simulink model "Cambers"  (R2024b)
settings: Solver=VariableStepAuto  StartTime=0  StopTime=30  RelTol=1e-3
libraries: simulink x2
settings Model: Creator=owen  LastModifiedBy=owen

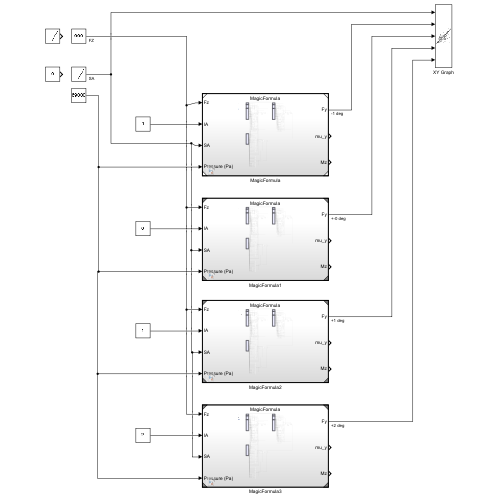
[thumbnail: Simulink's stored preview of the top-level diagram]
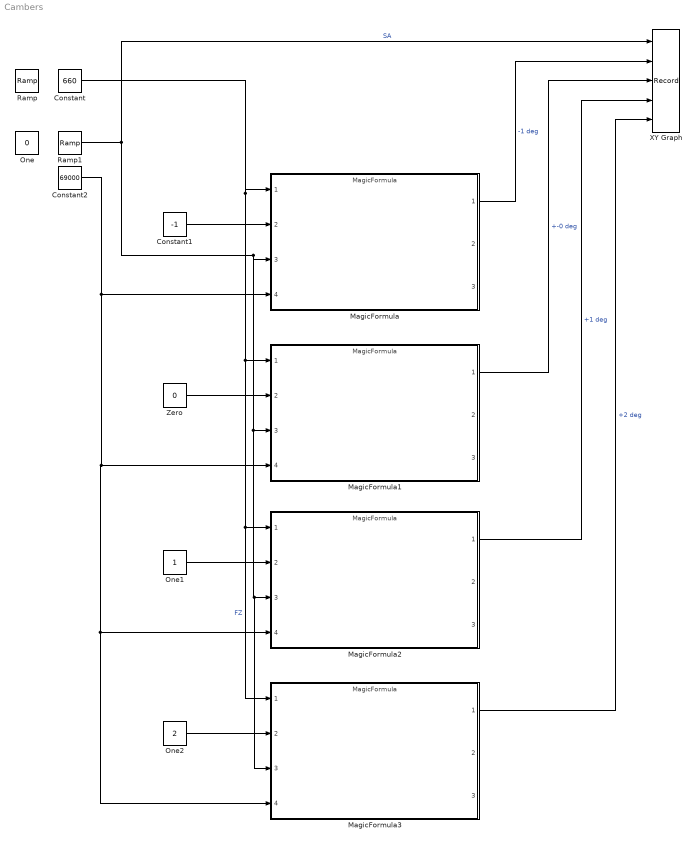
== system Cambers ==
  Constant : Constant  Value=660
  Constant1 : Constant  Value=-1
  Constant2 : Constant  Value=69000
  MagicFormula{,1..3} (4 alike) : ModelReference  ModelNameDialog=MagicFormula.slx  SimulationMode=Normal  ModelReferenceVersion=1.51
  One : Constant  Value=0  OutDataTypeStr=Inherit: Inherit via back propagation
  One1 : Constant  OutDataTypeStr=Inherit: Inherit via back propagation
  One2 : Constant  Value=2  OutDataTypeStr=Inherit: Inherit via back propagation
  Ramp : simulink/Sources/Ramp  slope=1  start=0  InitialOutput=0
  Ramp1 : simulink/Sources/Ramp  slope=1  start=0  InitialOutput=-15
  XY Graph : Record  FileSettingsInternal="{\"entries\":[{\"content\":{\"excelSettings\":{\"content\":{},\"type\":\"Streamout.ExcelSettings\"}},\"type\":\"Streamout.FileSettingStorage\",\"uuid\":\"\"}],\"packageUris\":[\"http:\\/\\/schema.mathworks.com\\/mf0\\/streamout_blocks\\/R2020a\"],\"version\":\"1.0\"}"  Layout=[1 1]  SignalsInternal="{\"entries\":[{\"content\":{\"signals\":[{\"content\":{\"blockPath\":[],\"dimensions\":[1],\"domain\":\"\",\"lineColor\":\"#a2142f\",\"plots\":[ 1 ],\"port\":1,\"sid\":[\"\"],\"signalID\":1,\"signalName\":\"SA\"},\"type\":\"RecordBlkView.Signal\",\"uuid\":\"\"},{\"content\":{\"blockPath\":[],\"dimensions\":[1],\"domain\":\"\",\"lineColor\":\"#139fff\",\"plots\":[ 1 ],\"port\":2,\"sid\":[\"\"],\"signalID\":2,\"signalName\":\"-1 deg\"},\"type\":\"RecordBlkView.Signal\",\"uuid\":\"\"},{\"content\":{\"blockPath\":[],\"dimensions\":[1],\"domain\":\"\",\"lineColor\":\"#ff6929\",\"lineWidth\":2,\"plots\":[ 1 ],\"port\":3,\"sid\":[\"\"],\"signalID\":3,\"signalName\":\"+-0 deg\"},\"type\":\"RecordBlkView.Signal\",\"uuid\":\"\"},{\"content\":{\"blockPath\":[],\"dimensions\":[1],\"domain\":\"\",\"lineColor\":\"#b746ff\",\"lineWidth\":2,\"plots\":[ 1 ],\"port\":4,\"sid\":[\"\"],\"signalID\":4,\"signalName\":\"+1 deg\"},\"type\":\"RecordBlkView.Signal\",\"uuid\":\"\"},{\"content\":{\"blockPath\":[],\"dimensions\":[1],\"domain\":\"\",\"lineColor\":\"#64d413\",\"lineWidth\":2,\"plots\":[ 1 ],\"port\":5,\"sid\":[\"\"],\"signalID\":5,\"signalName\":\"+2 deg\"},\"type\":\"RecordBlkView.Signal\",\"uuid\":\"\"}]},\"type\":\"RecordBlkView.InputSignals\",\"uuid\":\"\"}],\"packageUris\":[\"http:\\/\\/schema.mathworks.com\\/mf0\\/streamout_blocks\\/R2020a\"],\"version\":\"1.0\"}"  VisualizationBindings="{\"xyplotplugin\":{\"info\":[{\"series\":[{\"bindingParametersList\":[{\"parameter\":\"X-Axis\",\"signalID\":1,\"signalName\":\"SA\"},{\"parameter\":\"Y-Axis\",\"signalID\":2,\"signalName\":\"-1 deg\"}],\"seriesID\":0},{\"bindingParametersList\":[{\"parameter\":\"X-Axis\",\"signalID\":1,\"signalName\":\"SA\"},{\"parameter\":\"Y-Axis\",\"signalID\":3,\"signalName\":\"+-0 deg\"}],\"seriesID\":1},{\"bindingParametersList\":[{\"parameter\":\"X-Axis\",\"signalID\":1,\"signalName\":\"SA\"},{\"parameter\":\"Y-Axis\",\"signalID\":4,\"signalName\":\"+1 deg\"}],\"seriesID\":2},{\"bindingParametersList\":[{\"parameter\":\"X-Axis\",\"signalID\":1,\"signalName\":\"SA\"},{\"parameter\":\"Y-Axis\",\"signalID\":5,\"signalName\":\"+2 deg\"}],\"seriesID\":3}],\"subplotID\":1}]}}"  CompatibilityTag=XY
  Zero : Constant  Value=0  OutDataTypeStr=Inherit: Inherit via back propagation
  wires:
  Constant/1 -> MagicFormula3/1, MagicFormula2/1, MagicFormula1/1, MagicFormula/1  "FZ"
  Ramp1/1 -> XY Graph/1, MagicFormula3/3, MagicFormula2/3, MagicFormula1/3, MagicFormula/3  "SA"
  MagicFormula/1 -> XY Graph/2  "-1 deg"
  MagicFormula3/1 -> XY Graph/5  "+2 deg"
  MagicFormula2/1 -> XY Graph/4  "+1 deg"
  MagicFormula1/1 -> XY Graph/3  "+-0 deg"
  Constant1/1 -> MagicFormula/2
  Zero/1 -> MagicFormula1/2
  One1/1 -> MagicFormula2/2
  One2/1 -> MagicFormula3/2
  Constant2/1 -> MagicFormula1/4, MagicFormula3/4, MagicFormula2/4, MagicFormula/4
